simulink model "Controlador"  (R2025b)
settings: Solver=VariableStepAuto  StartTime=0.0  StopTime=15.0  MaxStep=0.1  RelTol=1e-3
undefined symbols (not defined in the file): DenK, h0, NumK
settings Model: Creator=NMB  LastModifiedBy=NMB

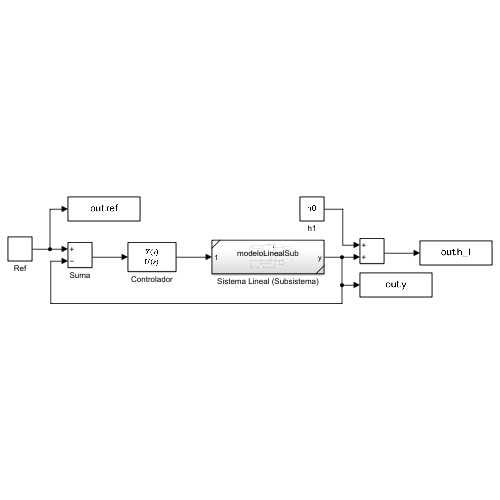
[thumbnail: Simulink's stored preview of the top-level diagram]
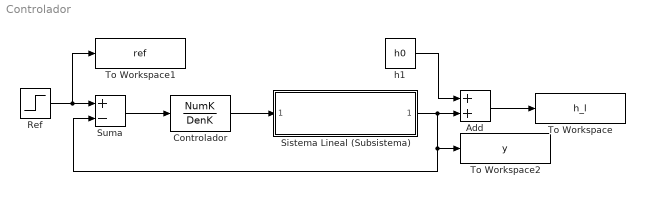
== system Controlador ==
  Add : Sum
  Controlador : TransferFcn  Numerator=NumK  Denominator=DenK
  Ref : Step  Time=5  After=0.4  SampleTime=0
  Sistema Lineal (Subsistema) : Subsystem  ReferencedSubsystem=modeloLinealSub
  Suma : Sum  Inputs=+-
  To Workspace : ToWorkspace  VariableName=h_l  SaveFormat=Timeseries  SampleTime=-1
  To Workspace1 : ToWorkspace  VariableName=ref  SaveFormat=Timeseries  SampleTime=-1
  To Workspace2 : ToWorkspace  VariableName=y  SaveFormat=Timeseries  SampleTime=-1
  h1 : Constant  Value=h0
  wires:
  Ref/1 -> To Workspace1/1, Suma/1
  Suma/1 -> Controlador/1
  Controlador/1 -> Sistema Lineal (Subsistema)/1
  Add/1 -> To Workspace/1
  h1/1 -> Add/1
  Sistema Lineal (Subsistema)/1 -> Suma/2, To Workspace2/1, Add/2
